simulink model "INVERTERCONTROL"  (R2022b)
settings: Solver=ode4  StartTime=0.0  StopTime=0.1  FixedStep=1e-6  RelTol=1e-3
values from neighbouring files (symbols this model uses):
  Iref = 11.96*sqrt(2)    [gridinverter.m]
  L = 2.4*10^-3    (= 0.0024)    [gridinverter.m]
  phiref = 0    [gridinverter.m]
  R = 1*10^-3    (= 0.001)    [gridinverter.m]
  Vgrid = 50*sqrt(2)    [gridinverter.m]
  Vpv = 80    [gridinverter.m]
libraries: spsMosfetLib x4, spsPowerLib x3, spsCurrentMeasurementLib x2, spsOnDelayLib x2, spsVoltageMeasurementLib x2, spsACVoltageSourceLib x1, spsDCVoltageSourceLib x1, simulink_extras x1, spsMeanLib x1, spsPLLLib x1, simulink x1, spsSeriesRLCBranchLib x1
settings Model: Creator=RYAN CHAN  LastModifiedBy=ZinouAb
settings DebuggingCC: UnconnectedInputMsg=warning  UnconnectedOutputMsg=warning  UnconnectedLineMsg=warning
settings ModelReferenceCC: EnableRefExpFcnMdlSchedulingChecks=on
settings RTWCC: DLArmComputeVersion=19.05

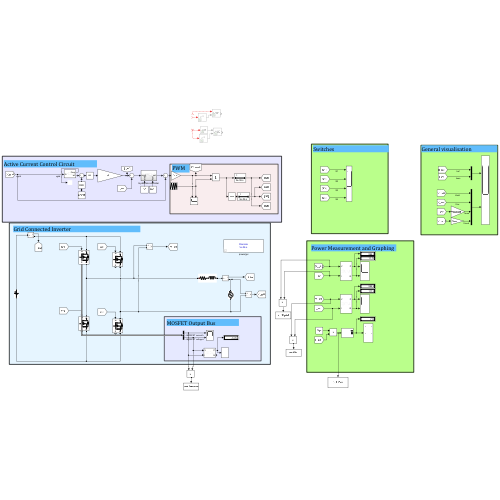
[thumbnail: Simulink's stored preview of the top-level diagram]
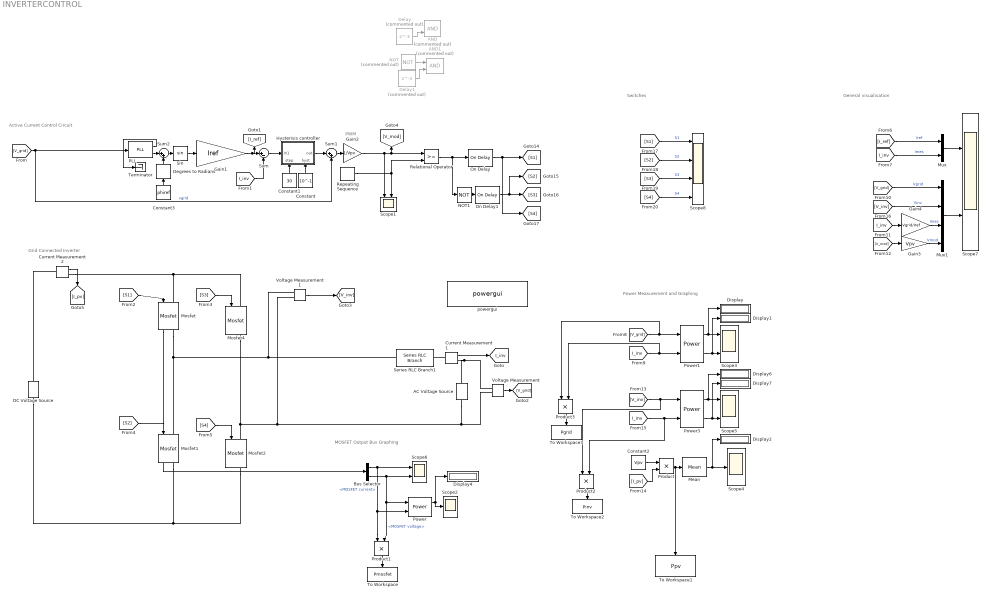
== system INVERTERCONTROL ==
  note: Active Current Control Circuit
  note: Grid Connected Inverter
  note: Power Measurement and Graphing
  note: PWM
  note: MOSFET Output Bus Graphing
  note: General visualisation
  note: Switches
  AC Voltage Source : spsACVoltageSourceLib/AC Voltage Source  Amplitude=Vgrid  Phase=0  Frequency=50  SampleTime=0  Measurements=None  BusType=swing  Pref=10e3  Qref=0  Qmin=-inf  Qmax=+inf
  AND : Logic  Commented=on  AllPortsSameDT=off  OutDataTypeStr=boolean
  AND1 : Logic  Commented=on  AllPortsSameDT=off  OutDataTypeStr=boolean
  Bus Selector : BusSelector  OutputSignals=MOSFET current,MOSFET voltage
  Constant : Constant  Value=10^-1
  Constant1 : Constant  Value=30
  Constant2 : Constant  Value=Vpv
  Constant3 : Constant  Value=phiref
  Current Measurement1 : spsCurrentMeasurementLib/Current Measurement  PhasorSimulation=off  OutputType=Complex  PSBequivalent=0
  Current Measurement2 : spsCurrentMeasurementLib/Current Measurement  PhasorSimulation=off  OutputType=Complex  PSBequivalent=0
  DC Voltage Source : spsDCVoltageSourceLib/DC Voltage Source  Amplitude=Vpv  Measurements=None
  Degrees to Radians : simulink_extras/Transformations/Degrees to Radians
  Delay : Delay  Commented=on  DelayLength=3  SampleTime=1e-6
  Delay1 : Delay  Commented=on  DelayLength=3  SampleTime=1e-6
  Display{,1..2,4,6..7} (6 alike) : Display
  Gain1 : Gain  Gain=Iref
  Gain2 : Gain  Gain=1/Vpv
  Gain3 : Gain  Gain=Vpv
  Gain4 : Gain  Gain=Vgrid/Iref
  Hysterisis controller : Subsystem
      settings: PortSchema="{\"entries\":[{\"content\":{\"sides\":[{\"content\":{\"connectorIds\":[\"In1\"]},\"type\":\"ConnectorPlacement.EquallySpacedRectSide\",\"uuid\":\"f66aa083-2ee8-4426-b441-0f8ce3c91bc6\"},{\"content\":{\"connectorIds\":[\"Out1\"],\"side\":\"RIGHT\"},\"type\":\"ConnectorPlacement.EquallySpacedRectSide\",\"uuid\":\"e535ff9d-11f2-429a-8d26-bff265e6dce4\"},{\"content\":{\"connectorIds\":[],\"side\":\"TOP\"},\"type\":\"ConnectorPlacement.EquallySpacedRectSide\",\"uuid\":\"3bf3f486-5ffc-4655-8aef-50265858aab1\"},{\"content\":{\"connectorIds\":[\"In2\",\"In3\"],\"side\":\"BOTTOM\"},\"type\":\"ConnectorPlacement.EquallySpacedRectSide\",\"uuid\":\"619b2421-7bbc-4c41-b693-a17d0c478cc9\"}]},\"type\":\"ConnectorPlacement.EquallySpacedConnector\",\"uuid\":\"4c23f3cf-154a-4c58-b671-46cc18db332d\"}],\"packageUris\":[\"http://schema.mathworks.com/mf0/Connector/R2020b\"],\"version\":\"1.0\"}"
  Mean : spsMeanLib/Mean  Freq=60  Vinit=0  Ts=0
  Mosfet{,1..2,4} (4 alike) : spsMosfetLib/Mosfet  Ron=0.27  Lon=0  Rd=0.01  Vfd=1.1  IC=0  Rs=1e5  Cs=inf  Measurements=on
  Mux : Mux  Inputs=2
  Mux1 : Mux
  NOT : Logic  Commented=on  Operator=NOT  AllPortsSameDT=off  OutDataTypeStr=boolean
  NOT1 : Logic  Operator=NOT  AllPortsSameDT=off  OutDataTypeStr=boolean
  On Delay : spsOnDelayLib/On Delay  DelayType=On delay  delay=delay  ic=0  Ts=0
  On Delay1 : spsOnDelayLib/On Delay  DelayType=On delay  delay=delay  ic=0  Ts=0
  PLL : spsPLLLib/PLL  Fmin=45  Par_Init=[0, 50]  ParK=[180, 3200, 1]  TcD=162e-6  MaxRateChangeFreq=12  FilterCutOffFreq=25  Ts=0  AGC=on
  Power : spsPowerLib/Power  Freq=50  Vinit=[1, 0]  Iinit=[1, 0]  Ts=0
  Power1 : spsPowerLib/Power  Freq=50  Vinit=[1, 0]  Iinit=[1, 0]  Ts=0
  Power3 : spsPowerLib/Power  Freq=50  Vinit=[1, 0]  Iinit=[1, 0]  Ts=0
  Product{,1..3} (4 alike) : Product
  Relational Operator : RelationalOperator  OutDataTypeStr=boolean  RndMeth=Simplest  InputSameDT=off
  Repeating Sequence : simulink/Sources/Repeating Sequence  rep_seq_t=[0 0.5e-4 1e-4]  rep_seq_y=[-1 1 -1]
  Scope{1,3,5..7} (5 alike) : Scope  NumInputPorts=2
  Scope2 : Scope
  Scope4 : Scope
  Scope8 : Scope  NumInputPorts=4
  Series RLC Branch1 : spsSeriesRLCBranchLib/Series RLC Branch  LConnTagsString=__new0  RConnTagsString=__new0  BranchType=RL  Resistance=R  Inductance=L  SetiL0=off  InitialCurrent=0  Capacitance=1e-6  Setx0=off  InitialVoltage=0  Measurements=None
  Sin : Trigonometry
  Sum : Sum  Inputs=|+-
  Sum1 : Sum  Inputs=|++
  Sum2 : Sum  Inputs=|++
  Terminator : Terminator
  To Workspace : ToWorkspace  VariableName=Pmosfet  SaveFormat=Timeseries  SampleTime=-1
  To Workspace1 : ToWorkspace  VariableName=Ppv  SaveFormat=Timeseries  SampleTime=-1
  To Workspace2 : ToWorkspace  VariableName=Pinv  SaveFormat=Timeseries  SampleTime=-1
  To Workspace3 : ToWorkspace  VariableName=Pgrid  SaveFormat=Timeseries  SampleTime=-1
  Voltage Measurement : spsVoltageMeasurementLib/Voltage Measurement  PhasorSimulation=off  OutputType=Complex  PSBequivalent=0
  Voltage Measurement1 : spsVoltageMeasurementLib/Voltage Measurement  PhasorSimulation=off  OutputType=Complex  PSBequivalent=0
  powergui : spspowerguiLib/powergui  Priority=1  SimulationMode=Discrete  SampleTime=1e-6  frequency=60  Iterations=50  frequencyindice=50  Pbase=100e6  ErrMax=1e-4  UnitsV=kV  UnitsW=MW  buscounter=0  FunctionMessages=off  echomessages=off  EnableUseOfTLC=off  CurrentSourceSwitches=off  DisableSnubberDevices=off  DisableRonSwitches=off  DisableVfSwitches=off  DisplayEquations=off  AutomaticDiscreteSolvers=off  SolverType=Tustin/Backward Euler (TBE)  Interpol=off  ExternalGateDelay=off  methode=off  Ts=100  x0status=blocks  SPID=on  SwTol=0  HookPort=off  NonlinearTolerance=1e-4  nMaxIteration=100  ContinueOnMaxIteration=off  RestoreLinks=warning  ResistiveCurrentMeasurement=off  Frange=[0:2:500]  Ylog=off  Xlog=on  ShowGrid=off  save=off  variable=ZData  structure=0  ZoomFFT=off  StartTime=0.0  cycles=1  DisplayStyle=1  fundamental=60  FreqAxis=off  MaxFrequency=1000  frequencyindicesteady=1  RmsSteady=1  display=off
  tag scope: I_inv=global
  wires:
  [V_grid] -> PLL/1, Sum1/2  "vgrid"
  Sin/1 -> Gain1/1
  Gain1/1 -> Sum/1, [I_ref]
  Sum/1 -> Hysterisis controller/1(In1)
  Hysterisis controller/1(out) -> Sum1/1
  Sum1/1 -> Gain2/1
  Repeating Sequence/1 -> Relational Operator/2, Scope1/2
  Current Measurement1/1 -> [I_inv]
  [S3] -> Mosfet4/1
  [S1] -> Mosfet/1
  Voltage Measurement/1 -> [V_grid]
  [S2] -> Mosfet1/1
  [S4] -> Mosfet2/1
  PLL/2 -> Sum2/1
  PLL/1 -> Terminator/1
  Voltage Measurement1/1 -> [V_inv]
  [I_inv] -> Sum/2
  Constant1/1 -> Hysterisis controller/2(step)
  Constant/1 -> Hysterisis controller/3(hyst)
  Bus Selector/1 -> Product1/1, Power/2, Scope6/1  "<MOSFET current>"
  Bus Selector/2 -> Product1/2, Power/1, Scope6/2  "<MOSFET voltage>"
  Mosfet/1 -> Bus Selector/1
  Mux/1 -> Scope7/1
  [I_ref] -> Mux/1  "Iref"
  [I_inv] -> Mux/2  "Imes"
  Gain2/1 -> [V_mod], Relational Operator/1, Scope1/1
  [V_mod] -> Gain3/1
  [I_inv] -> Gain4/1
  [V_grid] -> Mux1/1  "Vgrid"
  Gain3/1 -> Mux1/4  "Vmod"
  Mux1/1 -> Scope7/2
  Power1/1 -> Display/1, Scope3/1
  Power1/2 -> Display1/1, Scope3/2
  Constant2/1 -> Product/1
  [I_pv] -> Product/2
  Current Measurement2/1 -> [I_pv]
  Gain4/1 -> Mux1/3  "Imes"
  Power/1 -> Display4/1, Scope2/1
  Power3/2 -> Display7/1, Scope5/2
  Power3/1 -> Display6/1, Scope5/1
  [V_inv] -> Mux1/2  "Vinv"
  Sum2/1 -> Sin/1
  Degrees to Radians/1 -> Sum2/2
  Constant3/1 -> Degrees to Radians/1
  Mean/1 -> Scope4/1, Display2/1
  [S1] -> Scope8/1  "S1"
  [S2] -> Scope8/2  "S2"
  [S3] -> Scope8/3  "S3"
  [S4] -> Scope8/4  "S4"
  Relational Operator/1 -> NOT1/1, On Delay/1
  On Delay1/1 -> [S2], [S3]
  NOT/1 -> AND1/1
  Delay/1 -> AND/2
  ? -> Delay/1
  ? -> Delay1/1
  Delay1/1 -> AND1/2
  ? -> AND/1
  ? -> NOT/1
  On Delay/1 -> [S4], [S1]
  NOT1/1 -> On Delay1/1
  Product1/1 -> To Workspace/1
  Product/1 -> To Workspace1/1, Mean/1
  [V_inv] -> Product2/1, Power3/1
  [I_inv] -> Product2/2, Power3/2
  Product2/1 -> To Workspace2/1
  [I_inv] -> Product3/2, Power1/2
  Product3/1 -> To Workspace3/1
  [V_grid] -> Product3/1, Power1/1
  connections:
  Voltage Measurement/LConn2 -- AC Voltage Source/LConn1 -- Voltage Measurement1/LConn2 -- Mosfet2/LConn1 -- Mosfet4/RConn1
  Voltage Measurement/LConn1 -- Current Measurement1/RConn1 -- AC Voltage Source/RConn1
  DC Voltage Source/LConn1 -- Mosfet2/RConn1 -- Mosfet1/RConn1
  Voltage Measurement1/LConn1 -- Series RLC Branch1/LConn1 -- Mosfet/RConn1 -- Mosfet1/LConn1
  Mosfet/LConn1 -- Current Measurement2/RConn1 -- Mosfet4/LConn1
  Current Measurement1/LConn1 -- Series RLC Branch1/RConn1
  DC Voltage Source/RConn1 -- Current Measurement2/LConn1

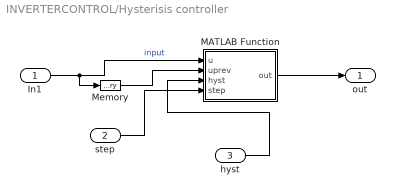
== system INVERTERCONTROL/Hysterisis controller ==
  In1 : Inport
  step : Inport  Port=2
  hyst : Inport  Port=3
  MATLAB Function : MATLAB Function  TreatAsAtomicUnit=on
  Memory : Memory
  out : Outport
  wires:
  In1/1 -> MATLAB Function/1(u), Memory/1  "input"
  Memory/1 -> MATLAB Function/2(uprev)
  MATLAB Function/1(out) -> out/1
  step/1 -> MATLAB Function/4(step)
  hyst/1 -> MATLAB Function/3(hyst)

== matlab function INVERTERCONTROL/Hysterisis controller/MATLAB Function ==
  data: u input; out output; uprev input; hyst input; step input
function out = hystcontrol(u,uprev,hyst,step)

if u>hyst
    out= uprev+step;
elseif u<hyst
    out= uprev-step;
else
    out=uprev;

end
